simulink model "qr_loops"  (Simulink 7.5)
settings: Solver=ode45  StartTime=0.0  StopTime=10.0  RelTol=1e-3
undefined symbols (not defined in the file): K, Ka, Kad, Kv, Ts
settings Model: Creator=jporter  LastModifiedBy=jporter

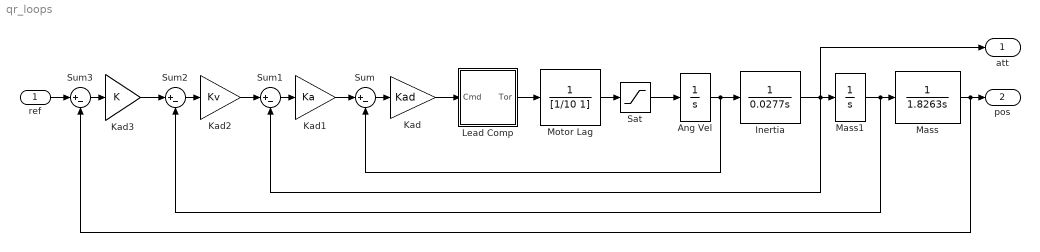
== system qr_loops ==
  ref : Inport  PortDimensions=1  DataType=single  OutDataTypeStr=single
  Ang Vel : TransferFcn  Denominator=[1 0]
  Inertia : TransferFcn  Denominator=[0.0277 0]
  Kad : Gain  Gain=Kad  ParameterDataTypeMode=single  ParameterDataType=sfix(16)  ParameterScaling=2^0  ParamDataTypeStr=single  OutDataType=sfix(16)  OutScaling=2^0
  Kad1 : Gain  Gain=Ka  ParameterDataTypeMode=single  ParameterDataType=sfix(16)  ParameterScaling=2^0  ParamDataTypeStr=single  OutDataType=sfix(16)  OutScaling=2^0
  Kad2 : Gain  Gain=Kv  ParameterDataTypeMode=single  ParameterDataType=sfix(16)  ParameterScaling=2^0  ParamDataTypeStr=single  OutDataType=sfix(16)  OutScaling=2^0
  Kad3 : Gain  Gain=K  ParameterDataTypeMode=single  ParameterDataType=sfix(16)  ParameterScaling=2^0  ParamDataTypeStr=single  OutDataType=sfix(16)  OutScaling=2^0
  Lead Comp : Subsystem
  Mass : TransferFcn  Denominator=[1.8263 0]
  Mass1 : TransferFcn  Denominator=[1 0]
  Motor Lag : TransferFcn  Denominator=[1/10 1]
  Sat : Saturate  UpperLimit=40  LowerLimit=-40  OutDataType=sfix(16)  OutScaling=2^0
  Sum{,1..3} (4 alike) : Sum  Inputs=|+-  OutDataType=sfix(16)  OutScaling=2^0
  att : Outport
  pos : Outport  Port=2
  wires:
  Motor Lag/1 -> Sat/1
  Sat/1 -> Ang Vel/1
  Inertia/1 -> att/1, Mass1/1, Sum1/2
  Mass/1 -> pos/1, Sum3/2
  Lead Comp/1(Tor) -> Motor Lag/1
  Ang Vel/1 -> Inertia/1, Sum/2
  Mass1/1 -> Mass/1, Sum2/2
  Sum/1 -> Kad/1
  Kad/1 -> Lead Comp/1(Cmd)
  Sum1/1 -> Kad1/1
  Sum2/1 -> Kad2/1
  Sum3/1 -> Kad3/1
  ref/1 -> Sum3/1
  Kad3/1 -> Sum2/1
  Kad2/1 -> Sum1/1
  Kad1/1 -> Sum/1

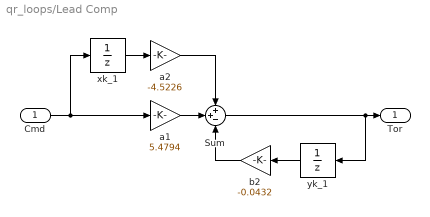
== system qr_loops/Lead Comp ==
  Cmd : Inport  PortDimensions=1  DataType=single  OutDataType=sfix(16)  OutScaling=2^0  OutDataTypeStr=single
  Sum : Sum  Inputs=++-  OutDataType=sfix(16)  OutScaling=2^0
  a1 : Gain  Gain=5.4794  ParameterDataTypeMode=single  ParameterDataType=sfix(16)  ParameterScaling=2^0  ParamDataTypeStr=single  OutDataType=sfix(16)  OutScaling=2^0
  a2 : Gain  Gain=-4.5226  ParameterDataTypeMode=single  ParameterDataType=sfix(16)  ParameterScaling=2^0  ParamDataTypeStr=single  OutDataType=sfix(16)  OutScaling=2^0
  b2 : Gain  Gain=-0.0432  ParameterDataTypeMode=single  ParameterDataType=sfix(16)  ParameterScaling=2^0  ParamDataTypeStr=single  OutDataType=sfix(16)  OutScaling=2^0
  xk_1 : UnitDelay  SampleTime=Ts
  yk_1 : UnitDelay  SampleTime=Ts
  Tor : Outport  OutDataType=sfix(16)  OutScaling=2^0
  wires:
  b2/1 -> Sum/3
  yk_1/1 -> b2/1
  Sum/1 -> Tor/1, yk_1/1
  a1/1 -> Sum/2
  a2/1 -> Sum/1
  xk_1/1 -> a2/1
  Cmd/1 -> xk_1/1, a1/1
